simulink model "example17and18"  (R2023b)
settings: Solver=VariableStepAuto  StartTime=0.0  StopTime=10.0  RelTol=1e-3
settings Model: Creator=ray  LastModifiedBy=ray

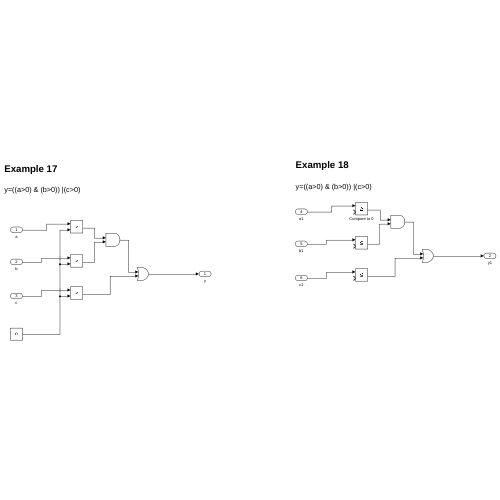
[thumbnail: Simulink's stored preview of the top-level diagram]
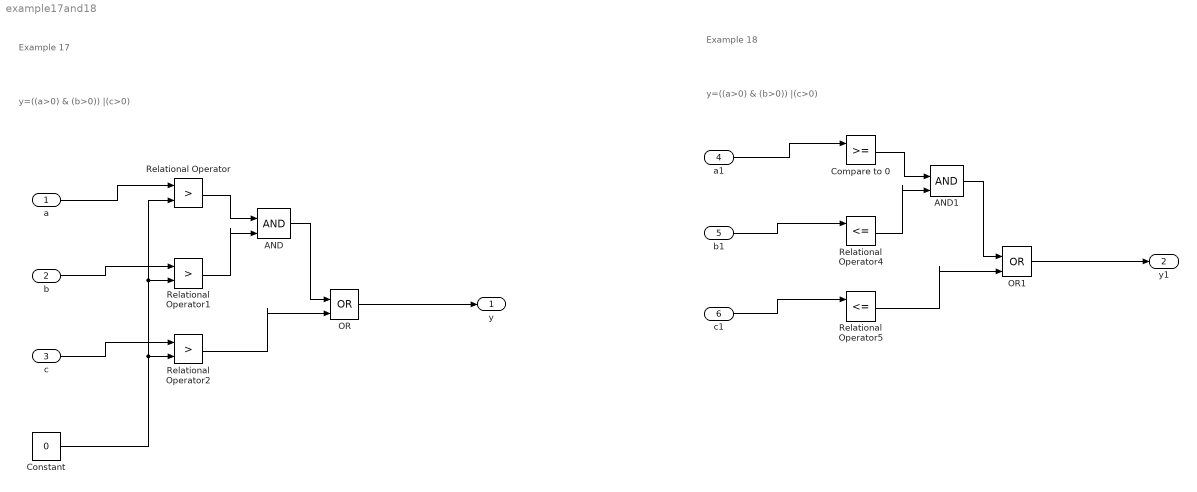
== system example17and18 ==
  note: y=((a>0) & (b>0)) |(c>0)
  note: Example 17
  note: y=((a>0) & (b>0)) |(c>0)
  note: Example 18
  a : Inport
  b : Inport  Port=2
  c : Inport  Port=3
  a1 : Inport  Port=4
  b1 : Inport  Port=5
  c1 : Inport  Port=6
  AND : Logic  IconShape=distinctive  AllPortsSameDT=off  OutDataTypeStr=boolean
  AND1 : Logic  IconShape=distinctive  AllPortsSameDT=off  OutDataTypeStr=boolean
  Compare to 0 : RelationalOperator  OutDataTypeStr=boolean  RndMeth=Simplest  InputSameDT=off
  Constant : Constant  Value=0
  OR : Logic  Operator=OR  IconShape=distinctive  AllPortsSameDT=off  OutDataTypeStr=boolean
  OR1 : Logic  Operator=OR  IconShape=distinctive  AllPortsSameDT=off  OutDataTypeStr=boolean
  Relational Operator : RelationalOperator  Operator=>  OutDataTypeStr=boolean  RndMeth=Simplest  InputSameDT=off
  Relational Operator1 : RelationalOperator  Operator=>  OutDataTypeStr=boolean  RndMeth=Simplest  InputSameDT=off
  Relational Operator2 : RelationalOperator  Operator=>  OutDataTypeStr=boolean  RndMeth=Simplest  InputSameDT=off
  Relational Operator4 : RelationalOperator  Operator=<=  OutDataTypeStr=boolean  RndMeth=Simplest  InputSameDT=off
  Relational Operator5 : RelationalOperator  Operator=<=  OutDataTypeStr=boolean  RndMeth=Simplest  InputSameDT=off
  y : Outport
  y1 : Outport  Port=2
  wires:
  a/1 -> Relational Operator/1
  Constant/1 -> Relational Operator2/2, Relational Operator1/2, Relational Operator/2
  c/1 -> Relational Operator2/1
  b/1 -> Relational Operator1/1
  Relational Operator1/1 -> AND/2
  Relational Operator/1 -> AND/1
  AND/1 -> OR/1
  Relational Operator2/1 -> OR/2
  OR/1 -> y/1
  OR1/1 -> y1/1
  b1/1 -> Relational Operator4/1
  Relational Operator4/1 -> AND1/2
  c1/1 -> Relational Operator5/1
  Compare to 0/1 -> AND1/1
  Relational Operator5/1 -> OR1/2
  AND1/1 -> OR1/1
  a1/1 -> Compare to 0/1
